simulink model "rfsocChannelizer"  (R2024a)
settings: Solver=FixedStepDiscrete  StartTime=0.0  StopTime=inf  RelTol=1e-3
InitFcn:
  | %% Polyphase Setup
  | fftsize = 512;
  | ntaps = 12;
  | vsize = 16;
  | pfb = dsp.Channelizer('NumFrequencyBands',fftsize,'NumTapsPerBand',ntaps);
  | 
  | coe = pfb.coeffs;
  | coe = coe.Numerator;
  | 
  | 
  | 
  | %% NCO Setup
  | rfsocChannelizerInit();
values from neighbouring files (symbols this model uses):
  Fo = 200.7e6    (= 200700000)    [rfsocChannelizerInit.m]
  Fs = 1/Ts    (= 5000000000)    [rfsocChannelizerInit.m]
  incrScale = (2^N)/Fs    (= 3.2768e-06)    [rfsocChannelizerInit.m]
  N = 14    [rfsocChannelizerInit.m]
libraries: dsphdlsigops2 x12, hdlsllib x9, simulink x8, simulink_need_slupdate x2, dspmathops x1, dsphdlfiltering2 x1, dspsrcs4 x1
Description:
  | libiioSDRPSP_filter_example
  | 
  | A simple example model to demonstrate the use of MATLAB I/O alongside
  | hardware/software co-design.
  | 
  | Implements AXI programmable gain and bypassable filters on the Tx and Rx
  | paths of the HDL DUT.
settings Model: DataTypeOverride=Off  ExtModeTrigDuration=100  Creator=mfornero  LastModifiedBy=versal
settings SolverCC: AlgebraicLoopSolver=TrustRegion  PositivePriorityOrder=on  MaxZcPerStep=1
settings DataIOCC: SaveOutput=off  ReturnWorkspaceOutputs=off  StateSaveName=tmp_raccel_xout  SignalLoggingName=tmp_raccel_logsout
settings OptimizationCC: BlockReduction=off  ConditionallyExecuteInputs=off  DefaultParameterBehavior=Inlined  EnhancedBackFolding=on  PassReuseOutputArgsAs=Individual arguments  ZeroExternalMemoryAtStartup=off  ZeroInternalMemoryAtStartup=off  EfficientMapNaN2IntZero=off  MaxStackSize=64  OptimizeBlockOrder=speed  DifferentSizesBufferReuse=on  OptimizationCustomize=off  EfficientTunableParamExpr=on
settings DebuggingCC: AlgebraicLoopMsg=error  SingleTaskRateTransMsg=error  ParameterTunabilityLossMsg=error  UnconnectedInputMsg=warning  UnconnectedOutputMsg=warning  UnconnectedLineMsg=warning  PregeneratedLibrarySubsystemCodeDiagnostic=none  StrictBusMsg=ErrorOnBusTreatedAsVector  SFUnexpectedBacktrackingDiag=warning  SFNoUnconditionalDefaultTransitionDiag=warning  SFExecutionAtInitializationDiag=none  ArithmeticOperatorsInVariantConditions=warning
settings HardwareCC: ProdBitPerPointer=32  ProdBitPerSizeT=32  ProdBitPerPtrDiffT=32  ProdLargestAtomicFloat=None  ProdIntDivRoundTo=Undefined  ProdEndianess=Unspecified  ProdWordSize=32  ProdHWDeviceType=ASIC/FPGA->ASIC/FPGA  TargetBitPerLong=64  TargetBitPerPointer=64  TargetBitPerSizeT=64  TargetBitPerPtrDiffT=64  TargetLongLongMode=on  TargetIntDivRoundTo=Zero  TargetEndianess=LittleEndian  TargetWordSize=64  TargetHWDeviceType=Custom Processor->MATLAB Host Computer  ProdEqTarget=off  HardwareBoardFeatureSet=SoCBlockset
settings ModelReferenceCC: EnableRefExpFcnMdlSchedulingChecks=on  ModelReferenceNumInstancesAllowed=Single
settings SFSimCC: SimUseLocalCustomCode=off  CustomCodeUndefinedFunction=UseInterfaceOnly
settings RTWCC: Description=Embedded Coder  SystemTargetFile=ert.tlc  HardwareBoard=Xilinx Zynq UltraScale+ RFSoC ZCU208 Evaluation Kit  TLCOptions="-aInlineSetEventsForThisBaseRateFcn=TLC_FALSE -aSuppressMultiTaskScheduler=TLC_FALSE  -aRateBasedStepFcn=0"  TemplateMakefile=ert_default_tmf  RTWVerbose=off  RTWUseLocalCustomCode=off  RTWUseSimCustomCode=on  Toolchain=Linaro AArch64 Linux v6.3.1  GPUComputeCapability=3.5  DLArmComputeVersion=19.05
settings CodeAppCC: ForceParamTrailComments=on  IgnoreCustomStorageClasses=off  MaxIdLength=128  OperatorAnnotations=on  SimulinkDataObjDesc=on  SFDataObjDesc=on  MangleLength=10  InsertBlockDesc=on
settings ERTTargetCC: InlinedParameterPlacement=NonHierarchical
settings ConfigComp: CovMetricSettings=dw  CovSaveCumulativeToWorkspaceVar=on  CovSaveSingleToWorkspaceVar=on  CovExternalEMLEnable=off

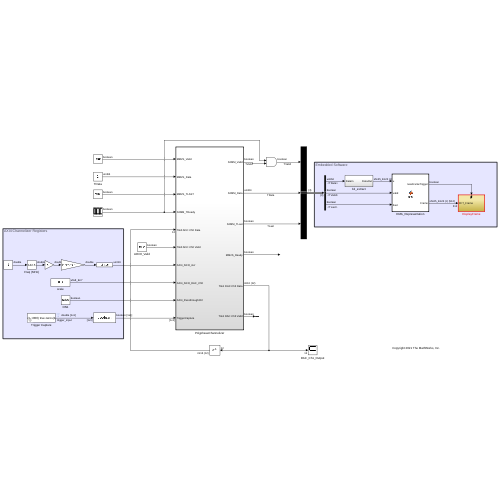
[thumbnail: Simulink's stored preview of the top-level diagram]
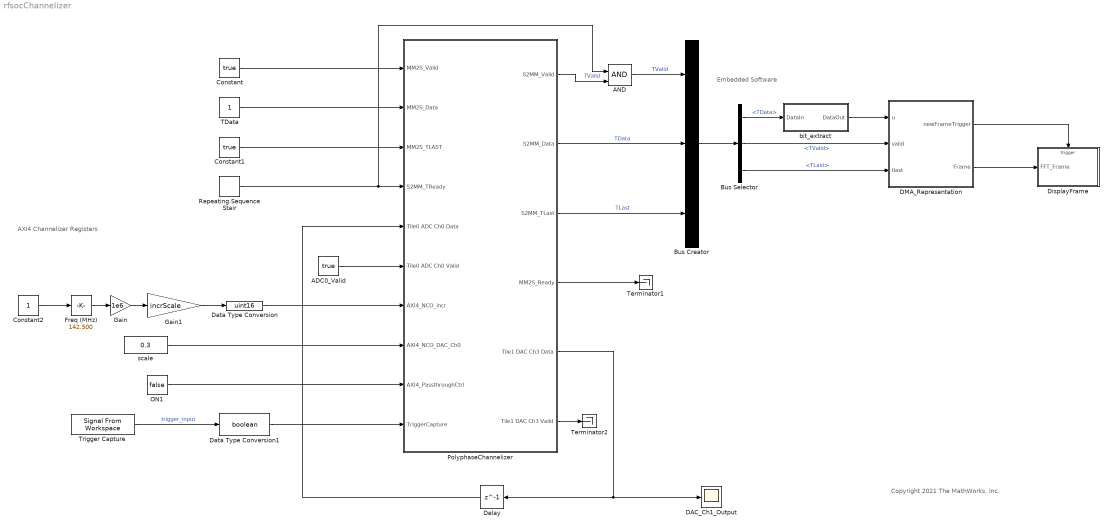
== system rfsocChannelizer ==
  note: AXI4 Channelizer Registers
  note: Embedded Software
  note: Copyright 2021 The MathWorks, Inc.
  ADC0_Valid : Constant  Value=true  SampleTime=-1
  AND : Logic  IconShape=distinctive  AllPortsSameDT=off  OutDataTypeStr=boolean
  Bus Creator : BusCreator  Inputs=3
  Bus Selector : BusSelector  OutputSignals=TData,TValid,TLast
  Constant : Constant  Value=true  SampleTime=1
  Constant1 : Constant  Value=true  SampleTime=-1
  Constant2 : Constant  SampleTime=1
  DAC_Ch1_Output : Scope
  DMA_Representation : MATLAB Function  TreatAsAtomicUnit=on
  Data Type Conversion : DataTypeConversion  OutDataTypeStr=uint16  SaturateOnIntegerOverflow=off  RndMeth=Floor
  Data Type Conversion1 : DataTypeConversion  OutDataTypeStr=boolean  SaturateOnIntegerOverflow=off  RndMeth=Floor
  Delay : Delay  DelayLength=1
  DisplayFrame : Subsystem
  Freq (MHz) : simulink/Math Operations/Slider Gain  gain=142.500  low=0  high=250
  Gain : Gain  Gain=1e6
  Gain1 : Gain  Gain=incrScale
  ON1 : Constant  Value=false  OutDataTypeStr=boolean  SampleTime=-1
  PolyphaseChannelizer : Subsystem  TreatAsAtomicUnit=on
  Repeating Sequence Stair : simulink/Sources/Repeating Sequence Stair  OutValues=[1 1 0 1 1 1 0 1 1]  tsamp=-1  OutMin=[]  OutMax=[]  OutDataTypeStr=fixdt('boolean')  OutputDataTypeScalingMode=Specify via dialog  OutDataType=fixdt('boolean')  ConRadixGroup=Best Precision: Vector-wise  OutScaling=[]
  TData : Constant  OutDataTypeStr=fixdt(0,64,0)  SampleTime=-1
  Terminator1 : Terminator
  Terminator2 : Terminator
  Trigger Capture : dspsrcs4/Signal From Workspace  X=[zeros(1,1000) true zeros(1,500)]  Ts=1  nsamps=1  OutputAfterFinalValue=Cyclic repetition  ignoreOrWarnInputAndFrameLengths=off  OutputFrames=off
  bit_extract : Subsystem
  scale : Constant  Value=0.3  OutDataTypeStr=fixdt(0,8,7)  SampleTime=-1
  wires:
  Constant/1 -> PolyphaseChannelizer/1(MM2S_Valid)
  TData/1 -> PolyphaseChannelizer/2(MM2S_Data)
  Gain/1 -> Gain1/1
  Freq (MHz)/1 -> Gain/1
  Constant2/1 -> Freq (MHz)/1
  Gain1/1 -> Data Type Conversion/1
  DMA_Representation/1(newFrameTrigger) -> DisplayFrame/Trigger
  DMA_Representation/2(Frame) -> DisplayFrame/1(FFT_Frame)
  bit_extract/1(DataOut) -> DMA_Representation/1(u)
  Constant1/1 -> PolyphaseChannelizer/3(MM2S_TLAST)
  PolyphaseChannelizer/4(MM2S_Ready) -> Terminator1/1
  Data Type Conversion/1 -> PolyphaseChannelizer/7(AXI4_NCO_incr)
  scale/1 -> PolyphaseChannelizer/8(AXI4_NCO_DAC_Ch0)
  ON1/1 -> PolyphaseChannelizer/9(AXI4_PassthroughCtrl)
  PolyphaseChannelizer/2(S2MM_Data) -> Bus Creator/2  "TData"
  PolyphaseChannelizer/3(S2MM_TLast) -> Bus Creator/3  "TLast"
  Bus Creator/1 -> Bus Selector/1
  Bus Selector/1 -> bit_extract/1(DataIn)  "<TData>"
  Bus Selector/2 -> DMA_Representation/2(valid)  "<TValid>"
  Bus Selector/3 -> DMA_Representation/3(tlast)  "<TLast>"
  ADC0_Valid/1 -> PolyphaseChannelizer/6(Tile0 ADC Ch0 Valid)
  PolyphaseChannelizer/6(Tile1 DAC Ch3 Valid) -> Terminator2/1
  PolyphaseChannelizer/5(Tile1 DAC Ch3 Data) -> Delay/1, DAC_Ch1_Output/1
  Trigger Capture/1 -> Data Type Conversion1/1  "trigger_input"
  Delay/1 -> PolyphaseChannelizer/5(Tile0 ADC Ch0 Data)
  Data Type Conversion1/1 -> PolyphaseChannelizer/10(TriggerCapture)
  PolyphaseChannelizer/1(S2MM_Valid) -> AND/2  "TValid"
  AND/1 -> Bus Creator/1  "TValid"
  Repeating Sequence Stair/1 -> AND/1, PolyphaseChannelizer/4(S2MM_TReady)

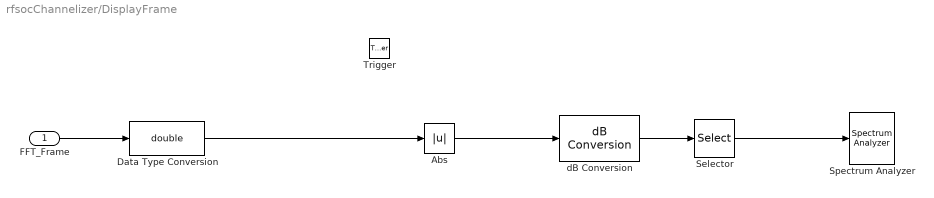
== system rfsocChannelizer/DisplayFrame ==
  FFT_Frame : Inport
  Trigger : TriggerPort  VariantControl=Variant
  Abs : Abs  SaturateOnIntegerOverflow=off
  Data Type Conversion : DataTypeConversion  OutDataTypeStr=double  SaturateOnIntegerOverflow=off  RndMeth=Floor
  Selector : Selector  InputPortWidth=512  IndexOptions=Index vector (dialog)  Indices=1:256  OutputSizes=1
  Spectrum Analyzer : SpectrumAnalyzer  WindowPosition=[613.000000,47.000000,1109.000000,792.000000,]  ScopeFrameLocation=window  InputDomain=Frequency  ViewType=Spectrum and spectrogram  SampleRateSource=Property  SampleRate=Fs  PlotAsTwoSidedSpectrum=off  AxesScaling=Manual  AveragingMethod=Exponential  SpectrumUnits=Auto  YLimits=[-140.0,0.1]  AllowFFTLengthLessThanSamplesPerUpdate=on  IsFrequencyInputMode=1
  dB Conversion : dspmathops/dB Conversion  dBtype=dB  intype=Amplitude  R=1  fuzz=on
  wires:
  FFT_Frame/1 -> Data Type Conversion/1
  dB Conversion/1 -> Selector/1
  Abs/1 -> dB Conversion/1
  Data Type Conversion/1 -> Abs/1
  Selector/1 -> Spectrum Analyzer/1

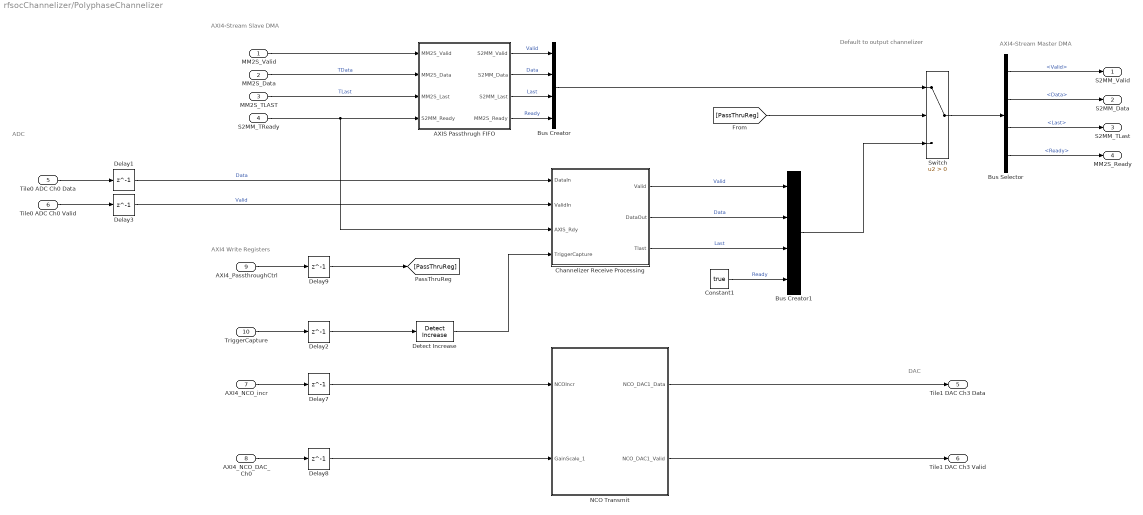
== system rfsocChannelizer/PolyphaseChannelizer ==
  note: Default to output channelizer
  note: DAC
  note: AXI4-Stream Slave DMA
  note: AXI4-Stream Master DMA
  note: AXI4 Write Registers
  note: ADC
  MM2S_Valid : Inport
  MM2S_Data : Inport  Port=2
  MM2S_TLAST : Inport  Port=3
  S2MM_TReady : Inport  Port=4
  Tile0 ADC Ch0 Data : Inport  Port=5
  Tile0 ADC Ch0 Valid : Inport  Port=6
  AXI4_NCO_incr : Inport  Port=7
  AXI4_NCO_DAC_Ch0 : Inport  Port=8
  AXI4_PassthroughCtrl : Inport  Port=9
  TriggerCapture : Inport  Port=10
  AXIS Passthrugh FIFO : Subsystem
  Bus Creator : BusCreator  Inputs=4
  Bus Creator1 : BusCreator  Inputs=4
  Bus Selector : BusSelector  OutputSignals=Valid,Data,Last,Ready
  "Channelizer Receive Processing " : Subsystem
  Constant1 : Constant  Value=true  OutDataTypeStr=boolean  SampleTime=-1
  Delay{1..3,7..9} (6 alike) : Delay  DelayLength=1
  Detect Increase : simulink/Logic and Bit Operations/Detect Increase  vinit=0.0  OutDataTypeStr=boolean
  NCO Transmit : Subsystem
  Switch : Switch  Criteria=u2 > Threshold  SaturateOnIntegerOverflow=off  InputSameDT=off
  S2MM_Valid : Outport  VectorParamsAs1DForOutWhenUnconnected=off
  S2MM_Data : Outport  Port=2  VectorParamsAs1DForOutWhenUnconnected=off
  S2MM_TLast : Outport  Port=3  VectorParamsAs1DForOutWhenUnconnected=off
  MM2S_Ready : Outport  Port=4  VectorParamsAs1DForOutWhenUnconnected=off
  Tile1 DAC Ch3 Data : Outport  Port=5
  Tile1 DAC Ch3 Valid : Outport  Port=6
  wires:
  Tile0 ADC Ch0 Data/1 -> Delay1/1
  Tile0 ADC Ch0 Valid/1 -> Delay3/1
  MM2S_Data/1 -> AXIS Passthrugh FIFO/2(MM2S_Data)  "TData"
  S2MM_TReady/1 -> AXIS Passthrugh FIFO/4(S2MM_Ready), "Channelizer Receive Processing "/3(AXIS_Rdy)
  "Channelizer Receive Processing "/3(Tlast) -> Bus Creator1/3  "Last"
  Bus Selector/4 -> MM2S_Ready/1  "<Ready>"
  AXI4_NCO_incr/1 -> Delay7/1
  AXI4_NCO_DAC_Ch0/1 -> Delay8/1
  NCO Transmit/1(NCO_DAC1_Data) -> Tile1 DAC Ch3 Data/1
  NCO Transmit/2(NCO_DAC1_Valid) -> Tile1 DAC Ch3 Valid/1
  MM2S_TLAST/1 -> AXIS Passthrugh FIFO/3(MM2S_Last)  "TLast"
  AXI4_PassthroughCtrl/1 -> Delay9/1
  Delay9/1 -> [PassThruReg]
  [PassThruReg] -> Switch/2
  "Channelizer Receive Processing "/2(DataOut) -> Bus Creator1/2  "Data"
  "Channelizer Receive Processing "/1(Valid) -> Bus Creator1/1  "Valid"
  Bus Creator1/1 -> Switch/3
  Bus Selector/1 -> S2MM_Valid/1  "<Valid>"
  Bus Selector/2 -> S2MM_Data/1  "<Data>"
  Bus Selector/3 -> S2MM_TLast/1  "<Last>"
  MM2S_Valid/1 -> AXIS Passthrugh FIFO/1(MM2S_Valid)
  AXIS Passthrugh FIFO/4(MM2S_Ready) -> Bus Creator/4  "Ready"
  AXIS Passthrugh FIFO/3(S2MM_Last) -> Bus Creator/3  "Last"
  AXIS Passthrugh FIFO/2(S2MM_Data) -> Bus Creator/2  "Data"
  AXIS Passthrugh FIFO/1(S2MM_Valid) -> Bus Creator/1  "Valid"
  Bus Creator/1 -> Switch/1
  Constant1/1 -> Bus Creator1/4  "Ready"
  Switch/1 -> Bus Selector/1
  Delay3/1 -> "Channelizer Receive Processing "/2(ValidIn)  "Valid"
  Delay1/1 -> "Channelizer Receive Processing "/1(DataIn)  "Data"
  Delay7/1 -> NCO Transmit/1(NCOIncr)
  Delay8/1 -> NCO Transmit/2(GainScale_1)
  TriggerCapture/1 -> Delay2/1
  Delay2/1 -> Detect Increase/1
  Detect Increase/1 -> "Channelizer Receive Processing "/4(TriggerCapture)

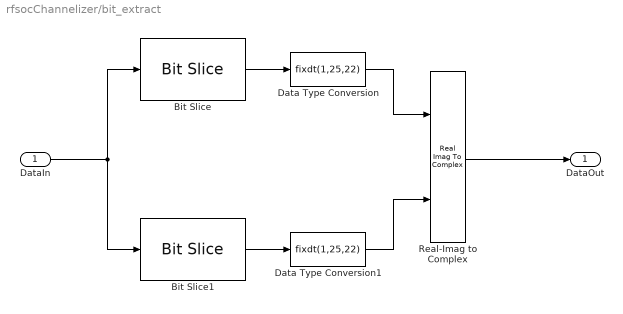
== system rfsocChannelizer/bit_extract ==
  DataIn : Inport
  Bit Slice : hdlsllib/Logic and Bit Operations/Bit Slice  lidx=49  ridx=25
  Bit Slice1 : hdlsllib/Logic and Bit Operations/Bit Slice  lidx=24  ridx=0
  Data Type Conversion : DataTypeConversion  OutDataTypeStr=fixdt(1,25,22)  ConvertRealWorld=Stored Integer (SI)  SaturateOnIntegerOverflow=off  RndMeth=Floor
  Data Type Conversion1 : DataTypeConversion  OutDataTypeStr=fixdt(1,25,22)  ConvertRealWorld=Stored Integer (SI)  SaturateOnIntegerOverflow=off  RndMeth=Floor
  Real-Imag to Complex : RealImagToComplex
  DataOut : Outport  VectorParamsAs1DForOutWhenUnconnected=off
  wires:
  DataIn/1 -> Bit Slice1/1, Bit Slice/1
  Bit Slice/1 -> Data Type Conversion/1
  Bit Slice1/1 -> Data Type Conversion1/1
  Data Type Conversion/1 -> Real-Imag to Complex/1
  Data Type Conversion1/1 -> Real-Imag to Complex/2
  Real-Imag to Complex/1 -> DataOut/1

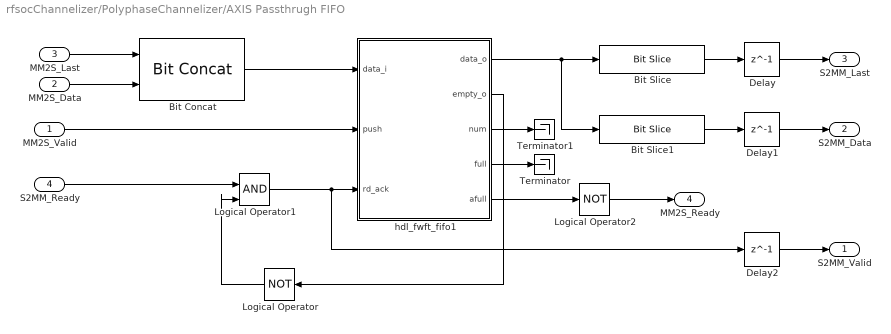
== system rfsocChannelizer/PolyphaseChannelizer/AXIS Passthrugh FIFO ==
  MM2S_Valid : Inport
  MM2S_Data : Inport  Port=2
  MM2S_Last : Inport  Port=3
  S2MM_Ready : Inport  Port=4
  Bit Concat : hdlsllib/Logic and Bit Operations/Bit Concat  numInputs=2
  Bit Slice : hdlsllib/Logic and Bit Operations/Bit Slice  lidx=64  ridx=64
  Bit Slice1 : hdlsllib/Logic and Bit Operations/Bit Slice  lidx=63  ridx=0
  Delay : Delay  DelayLength=1
  Delay1 : Delay  DelayLength=1
  Delay2 : Delay  DelayLength=1
  Logical Operator : Logic  Operator=NOT  IconShape=distinctive  AllPortsSameDT=off  OutDataTypeStr=boolean
  Logical Operator1 : Logic  IconShape=distinctive  AllPortsSameDT=off  OutDataTypeStr=boolean
  Logical Operator2 : Logic  Operator=NOT  IconShape=distinctive  AllPortsSameDT=off  OutDataTypeStr=boolean
  Terminator : Terminator
  Terminator1 : Terminator
  hdl_fwft_fifo1 : Subsystem  mask{FIFO_DEPTH=100, AFULL_THRESH=80}
      mask prompts: FIFO_DEPTH "FIFO Depth"; AFULL_THRESH "Almost Full Threshold"
      mask init:
      | FIFO_CNT_BITS=ceil(log2(FIFO_DEPTH+1+3));
  S2MM_Valid : Outport  VectorParamsAs1DForOutWhenUnconnected=off
  S2MM_Data : Outport  Port=2  VectorParamsAs1DForOutWhenUnconnected=off
  S2MM_Last : Outport  Port=3  VectorParamsAs1DForOutWhenUnconnected=off
  MM2S_Ready : Outport  Port=4  VectorParamsAs1DForOutWhenUnconnected=off
  wires:
  MM2S_Data/1 -> Bit Concat/2
  Bit Concat/1 -> hdl_fwft_fifo1/1(data_i)
  MM2S_Last/1 -> Bit Concat/1
  Logical Operator1/1 -> Delay2/1, hdl_fwft_fifo1/3(rd_ack)
  hdl_fwft_fifo1/2(empty_o) -> Logical Operator/1
  S2MM_Ready/1 -> Logical Operator1/1
  Bit Slice/1 -> Delay/1
  hdl_fwft_fifo1/1(data_o) -> Bit Slice1/1, Bit Slice/1
  Logical Operator/1 -> Logical Operator1/2
  hdl_fwft_fifo1/4(full) -> Terminator/1
  Delay2/1 -> S2MM_Valid/1
  Delay/1 -> S2MM_Last/1
  hdl_fwft_fifo1/3(num) -> Terminator1/1
  Delay1/1 -> S2MM_Data/1
  hdl_fwft_fifo1/5(afull) -> Logical Operator2/1
  Logical Operator2/1 -> MM2S_Ready/1
  Bit Slice1/1 -> Delay1/1
  MM2S_Valid/1 -> hdl_fwft_fifo1/2(push)

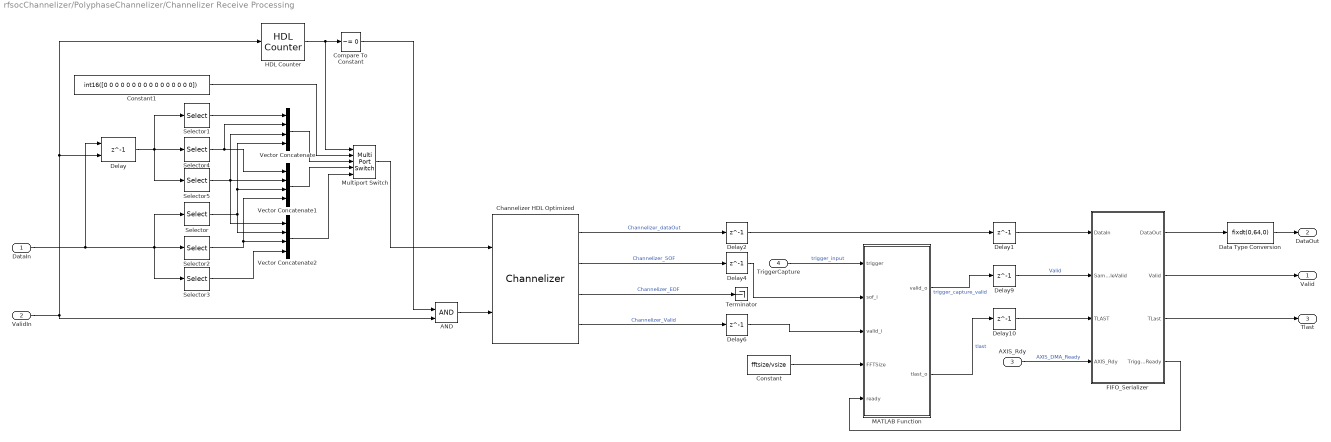
== system rfsocChannelizer/PolyphaseChannelizer/Channelizer Receive Processing  ==
  DataIn : Inport
  ValidIn : Inport  Port=2
  AXIS_Rdy : Inport  Port=3
  TriggerCapture : Inport  Port=4
  AND : Logic  IconShape=distinctive  AllPortsSameDT=off  OutDataTypeStr=boolean
  Channelizer HDL Optimized : dsphdlfiltering2/Channelizer  FilterCoefficients=pfb.coeffs.Numerator  FilterStructure=Direct form transposed  NumFrequencyBands=fftsize  ComplexMultiplication=Use 3 multipliers and 5 adders  Normalize=off  OutputSize=Same as input size  SimulateUsing=Code generation  roundingMode=Floor  overflowMode=off  CoefficientsDataTypeStr=Inherit: Same word length as input  FilterOutputDataTypeStr=Inherit: Same word length as input  ResetInputPort=off  StartOutputPort=on  EndOutputPort=on
  Compare To Constant : simulink/Logic and Bit Operations/Compare To Constant  relop=~=  const=0  OutDataTypeStr=boolean
  Constant : Constant  Value=fftsize/vsize  OutDataTypeStr=uint16  SampleTime=-1
  Constant1 : Constant  Value=int16([0 0 0 0 0 0 0 0 0 0 0 0 0 0 0 0])
  Data Type Conversion : DataTypeConversion  OutDataTypeStr=fixdt(0,64,0)  ConvertRealWorld=Stored Integer (SI)  SaturateOnIntegerOverflow=off  RndMeth=Floor
  Delay : Delay  DelayLength=1  InitialCondition=0  ShowEnablePort=on  UseCircularBuffer=on
      settings: InputPortMap=u0,e6
  Delay{1..2,4,6,9..10} (6 alike) : Delay  DelayLength=1
  FIFO_Serializer : Subsystem
  HDL Counter : hdlsllib/Sources/HDL Counter  CountType=Count limited  CountInit=0  CountStep=1  CountMax=3  CountFromType=Initial value  CountFrom=0  CountResetPort=off  CountLoadPort=off  CountEnbPort=on  CountDirPort=off  CountHitOutputPort=off  CountDataType=Unsigned  CountWordLen=2  CountFracLen=0  CountSampTime=1
  MATLAB Function : MATLAB Function  TreatAsAtomicUnit=on
  Multiport Switch : MultiPortSwitch  DataPortOrder=Zero-based contiguous  Inputs=4  zeroidx=on  SaturateOnIntegerOverflow=off  InputSameDT=off
  Selector : Selector  InputPortWidth=12  IndexOptions=Index vector (dialog)  Indices=[1 2 3 4]  OutputSizes=1
  Selector1 : Selector  InputPortWidth=12  IndexOptions=Index vector (dialog)  Indices=[1 2 3 4]  OutputSizes=1
  Selector2 : Selector  InputPortWidth=12  IndexOptions=Index vector (dialog)  Indices=[5 6 7 8]  OutputSizes=1
  Selector3 : Selector  InputPortWidth=12  IndexOptions=Index vector (dialog)  Indices=[9 10 11 12]  OutputSizes=1
  Selector4 : Selector  InputPortWidth=12  IndexOptions=Index vector (dialog)  Indices=[5 6 7 8]  OutputSizes=1
  Selector5 : Selector  InputPortWidth=12  IndexOptions=Index vector (dialog)  Indices=[9 10 11 12]  OutputSizes=1
  Terminator : Terminator
  Vector Concatenate : Concatenate  NumInputs=4
  Vector Concatenate1 : Concatenate  NumInputs=4
  Vector Concatenate2 : Concatenate  NumInputs=4
  Valid : Outport  VectorParamsAs1DForOutWhenUnconnected=off
  DataOut : Outport  Port=2  VectorParamsAs1DForOutWhenUnconnected=off
  Tlast : Outport  Port=3  VectorParamsAs1DForOutWhenUnconnected=off
  wires:
  Delay9/1 -> FIFO_Serializer/2(SampleValid)  "Valid"
  Delay10/1 -> FIFO_Serializer/3(TLAST)
  Delay1/1 -> FIFO_Serializer/1(DataIn)
  AXIS_Rdy/1 -> FIFO_Serializer/4(AXIS_Rdy)  "AXIS_DMA_Ready"
  FIFO_Serializer/1(DataOut) -> Data Type Conversion/1
  Data Type Conversion/1 -> DataOut/1
  FIFO_Serializer/2(Valid) -> Valid/1
  ValidIn/1 -> Delay/2, HDL Counter/1, AND/2
  Channelizer HDL Optimized/1 -> Delay2/1  "Channelizer_dataOut"
  Channelizer HDL Optimized/2 -> Delay4/1  "Channelizer_SOF"
  Channelizer HDL Optimized/3 -> Terminator/1  "Channelizer_EOF"
  Channelizer HDL Optimized/4 -> Delay6/1  "Channelizer_Valid"
  FIFO_Serializer/3(TLast) -> Tlast/1
  Constant/1 -> MATLAB Function/4(FFTSize)
  FIFO_Serializer/4(TriggerReady) -> MATLAB Function/5(ready)
  TriggerCapture/1 -> MATLAB Function/1(trigger)  "trigger_input"
  MATLAB Function/1(valid_o) -> Delay9/1  "trigger_capture_valid"
  Delay4/1 -> MATLAB Function/2(sof_i)
  Delay6/1 -> MATLAB Function/3(valid_i)
  MATLAB Function/2(tlast_o) -> Delay10/1  "tlast"
  Delay2/1 -> Delay1/1
  DataIn/1 -> Selector3/1, Selector2/1, Selector/1, Delay/1
  Delay/1 -> Selector4/1, Selector5/1, Selector1/1
  Selector1/1 -> Vector Concatenate/1
  Selector4/1 -> Vector Concatenate1/1, Vector Concatenate/2
  Selector5/1 -> Vector Concatenate2/1, Vector Concatenate1/2, Vector Concatenate/3
  Selector/1 -> Vector Concatenate1/3, Vector Concatenate/4, Vector Concatenate2/2
  Selector2/1 -> Vector Concatenate2/3, Vector Concatenate1/4
  Selector3/1 -> Vector Concatenate2/4
  Vector Concatenate/1 -> Multiport Switch/3
  Vector Concatenate1/1 -> Multiport Switch/4
  Vector Concatenate2/1 -> Multiport Switch/5
  Multiport Switch/1 -> Channelizer HDL Optimized/1
  HDL Counter/1 -> Compare To Constant/1, Multiport Switch/1
  Constant1/1 -> Multiport Switch/2
  AND/1 -> Channelizer HDL Optimized/2
  Compare To Constant/1 -> AND/1

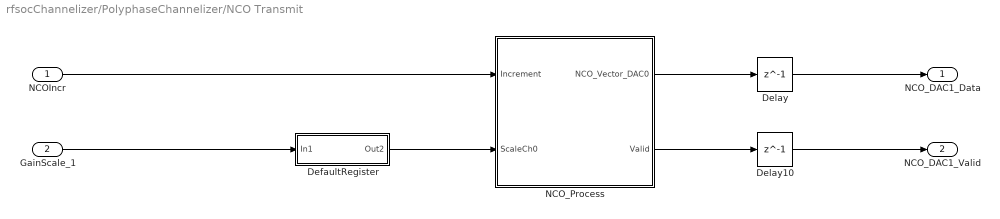
== system rfsocChannelizer/PolyphaseChannelizer/NCO Transmit ==
  NCOIncr : Inport
  GainScale_1 : Inport  Port=2
  DefaultRegister : Subsystem
  Delay : Delay  DelayLength=1
  Delay10 : Delay  DelayLength=1
  NCO_Process : Subsystem
  NCO_DAC1_Data : Outport  VectorParamsAs1DForOutWhenUnconnected=off
  NCO_DAC1_Valid : Outport  Port=2  VectorParamsAs1DForOutWhenUnconnected=off
  wires:
  Delay/1 -> NCO_DAC1_Data/1
  DefaultRegister/1(Out2) -> NCO_Process/2(ScaleCh0)
  NCO_Process/1(NCO_Vector_DAC0) -> Delay/1
  NCO_Process/2(Valid) -> Delay10/1
  NCOIncr/1 -> NCO_Process/1(Increment)
  GainScale_1/1 -> DefaultRegister/1(In1)
  Delay10/1 -> NCO_DAC1_Valid/1

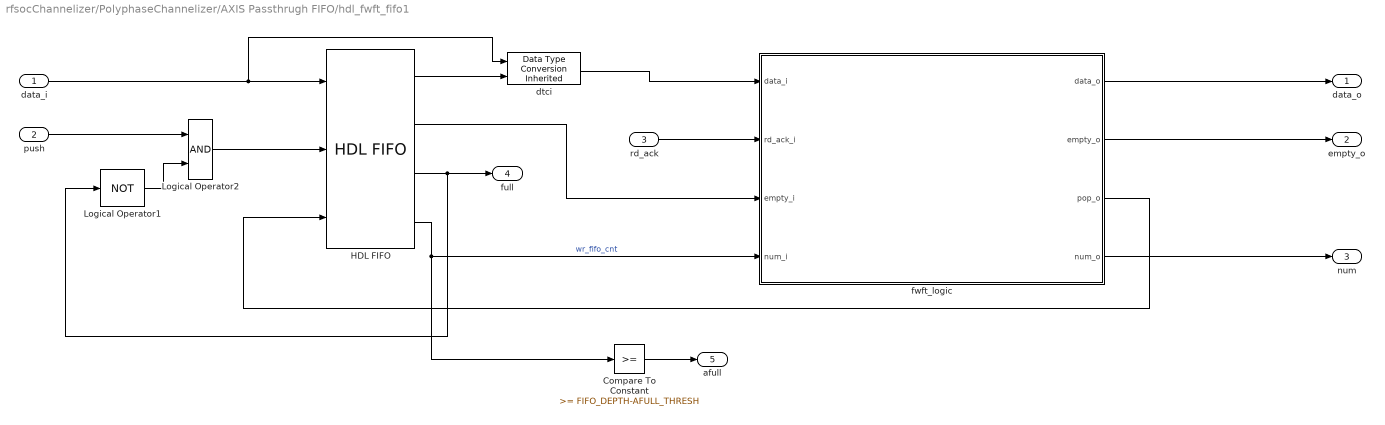
== system rfsocChannelizer/PolyphaseChannelizer/AXIS Passthrugh FIFO/hdl_fwft_fifo1 ==
  data_i : Inport
  push : Inport  Port=2
  rd_ack : Inport  Port=3
  Compare To Constant : simulink/Logic and Bit Operations/Compare To Constant  relop=>=  const=FIFO_DEPTH-AFULL_THRESH  OutDataTypeStr=boolean
  HDL FIFO : hdlsllib/HDL RAMs/HDL FIFO  fifo_size=FIFO_DEPTH  mode=Classic  ratio=1  push_msg=Error  pop_msg=Ignore  show_empty=on  show_full=on  show_num=on  LabelModeActiveChoice_Mode=Classic  rst_port=off
  Logical Operator1 : Logic  Operator=NOT  IconShape=distinctive  AllPortsSameDT=off  OutDataTypeStr=boolean
  Logical Operator2 : Logic  IconShape=distinctive  AllPortsSameDT=off  OutDataTypeStr=boolean
  dtci : simulink/Signal Attributes/Data Type Conversion Inherited  ConvertRealWorld=Real World Value  DoSatur=off
  fwft_logic : Subsystem
  data_o : Outport  VectorParamsAs1DForOutWhenUnconnected=off
  empty_o : Outport  Port=2  VectorParamsAs1DForOutWhenUnconnected=off
  num : Outport  Port=3  VectorParamsAs1DForOutWhenUnconnected=off
  full : Outport  Port=4  VectorParamsAs1DForOutWhenUnconnected=off
  afull : Outport  Port=5  VectorParamsAs1DForOutWhenUnconnected=off
  wires:
  Compare To Constant/1 -> afull/1
  fwft_logic/1(data_o) -> data_o/1
  HDL FIFO/2 -> fwft_logic/3(empty_i)
  rd_ack/1 -> fwft_logic/2(rd_ack_i)
  fwft_logic/2(empty_o) -> empty_o/1
  data_i/1 -> dtci/1, HDL FIFO/1
  fwft_logic/3(pop_o) -> HDL FIFO/3
  push/1 -> Logical Operator2/1
  Logical Operator2/1 -> HDL FIFO/2
  Logical Operator1/1 -> Logical Operator2/2
  HDL FIFO/1 -> dtci/2
  dtci/1 -> fwft_logic/1(data_i)
  HDL FIFO/3 -> Logical Operator1/1, full/1
  HDL FIFO/4 -> Compare To Constant/1, fwft_logic/4(num_i)  "wr_fifo_cnt"
  fwft_logic/4(num_o) -> num/1

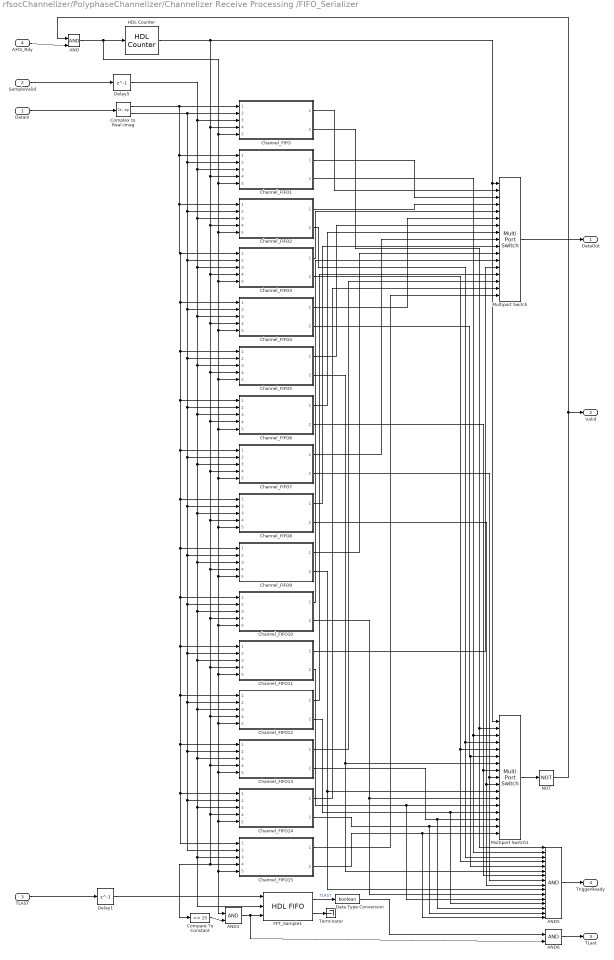
== system rfsocChannelizer/PolyphaseChannelizer/Channelizer Receive Processing /FIFO_Serializer ==
  DataIn : Inport
  SampleValid : Inport  Port=2
  TLAST : Inport  Port=3
  AXIS_Rdy : Inport  Port=4
  AND : Logic  IconShape=distinctive  AllPortsSameDT=off  OutDataTypeStr=boolean
  AND1 : Logic  IconShape=distinctive  AllPortsSameDT=off  OutDataTypeStr=boolean
  AND5 : Logic  Inputs=16  IconShape=distinctive  AllPortsSameDT=off  OutDataTypeStr=boolean
  AND6 : Logic  IconShape=distinctive  AllPortsSameDT=off  OutDataTypeStr=boolean
  Channel_FIFO : Subsystem  ReferencedSubsystem=Channel_FIFO  Index=0
  Channel_FIFO1 : Subsystem  ReferencedSubsystem=Channel_FIFO  Index=1
  Channel_FIFO10 : Subsystem  ReferencedSubsystem=Channel_FIFO  Index=10
  Channel_FIFO11 : Subsystem  ReferencedSubsystem=Channel_FIFO  Index=11
  Channel_FIFO12 : Subsystem  ReferencedSubsystem=Channel_FIFO  Index=12
  Channel_FIFO13 : Subsystem  ReferencedSubsystem=Channel_FIFO  Index=13
  Channel_FIFO14 : Subsystem  ReferencedSubsystem=Channel_FIFO  Index=14
  Channel_FIFO15 : Subsystem  ReferencedSubsystem=Channel_FIFO  Index=15
  Channel_FIFO2 : Subsystem  ReferencedSubsystem=Channel_FIFO  Index=2
  Channel_FIFO3 : Subsystem  ReferencedSubsystem=Channel_FIFO  Index=3
  Channel_FIFO4 : Subsystem  ReferencedSubsystem=Channel_FIFO  Index=4
  Channel_FIFO5 : Subsystem  ReferencedSubsystem=Channel_FIFO  Index=5
  Channel_FIFO6 : Subsystem  ReferencedSubsystem=Channel_FIFO  Index=6
  Channel_FIFO7 : Subsystem  ReferencedSubsystem=Channel_FIFO  Index=7
  Channel_FIFO8 : Subsystem  ReferencedSubsystem=Channel_FIFO  Index=8
  Channel_FIFO9 : Subsystem  ReferencedSubsystem=Channel_FIFO  Index=9
  Compare To Constant : simulink/Logic and Bit Operations/Compare To Constant  relop===  const=15  OutDataTypeStr=boolean
  Complex to Real-Imag : ComplexToRealImag
  Data Type Conversion : DataTypeConversion  OutDataTypeStr=boolean  SaturateOnIntegerOverflow=off  RndMeth=Floor
  Delay1 : Delay  DelayLength=1
  Delay5 : Delay  DelayLength=1
  FFT_Sample1 : hdlsllib/HDL RAMs/HDL FIFO  fifo_size=128  mode=FWFT  ratio=1  push_msg=Warning  pop_msg=Warning  show_empty=on  show_full=off  show_num=off  LabelModeActiveChoice_Mode=FWFT  rst_port=off
  HDL Counter : hdlsllib/Sources/HDL Counter  CountType=Count limited  CountInit=0  CountStep=1  CountMax=15  CountFromType=Initial value  CountFrom=0  CountResetPort=off  CountLoadPort=off  CountEnbPort=on  CountDirPort=off  CountHitOutputPort=off  CountDataType=Unsigned  CountWordLen=4  CountFracLen=0  CountSampTime=1
  Multiport Switch : MultiPortSwitch  DataPortOrder=Zero-based contiguous  Inputs=16  zeroidx=on  SaturateOnIntegerOverflow=off  InputSameDT=off
  Multiport Switch1 : MultiPortSwitch  DataPortOrder=Zero-based contiguous  Inputs=16  zeroidx=on  SaturateOnIntegerOverflow=off  InputSameDT=off
  NOT : Logic  Operator=NOT  IconShape=distinctive  AllPortsSameDT=off  OutDataTypeStr=boolean
  Terminator : Terminator
  DataOut : Outport  VectorParamsAs1DForOutWhenUnconnected=off
  Valid : Outport  Port=2  VectorParamsAs1DForOutWhenUnconnected=off
  TLast : Outport  Port=3  VectorParamsAs1DForOutWhenUnconnected=off
  TriggerReady : Outport  Port=4
  wires:
  AND1/1 -> AND6/2, FFT_Sample1/3
  Channel_FIFO2/1 -> Multiport Switch/4
  Compare To Constant/1 -> AND1/2
  DataIn/1 -> Complex to Real-Imag/1
  Data Type Conversion/1 -> AND6/1
  Channel_FIFO2/2 -> AND5/3, Multiport Switch1/4
  Channel_FIFO/1 -> Multiport Switch/2
  Multiport Switch/1 -> DataOut/1
  TLAST/1 -> Delay1/1
  Channel_FIFO1/1 -> Multiport Switch/3
  NOT/1 -> AND/1, Valid/1
  FFT_Sample1/1 -> Data Type Conversion/1  "TLAST"
  Channel_FIFO1/2 -> AND5/2, Multiport Switch1/3
  AXIS_Rdy/1 -> AND/2
  SampleValid/1 -> Delay5/1
  AND6/1 -> TLast/1
  Channel_FIFO/2 -> AND5/1, Multiport Switch1/2
  AND5/1 -> TriggerReady/1
  Channel_FIFO3/2 -> AND5/4, Multiport Switch1/5
  Multiport Switch1/1 -> NOT/1
  Channel_FIFO3/1 -> Multiport Switch/5
  Complex to Real-Imag/1 -> Channel_FIFO1/1, Channel_FIFO2/1, Channel_FIFO3/1, Channel_FIFO4/1, Channel_FIFO5/1, Channel_FIFO6/1, Channel_FIFO7/1, Channel_FIFO8/1, Channel_FIFO9/1, Channel_FIFO10/1, Channel_FIFO11/1, Channel_FIFO12/1, Channel_FIFO13/1, Channel_FIFO14/1, Channel_FIFO15/1, Channel_FIFO/1
  Complex to Real-Imag/2 -> Channel_FIFO1/2, Channel_FIFO2/2, Channel_FIFO3/2, Channel_FIFO4/2, Channel_FIFO5/2, Channel_FIFO6/2, Channel_FIFO7/2, Channel_FIFO8/2, Channel_FIFO9/2, Channel_FIFO10/2, Channel_FIFO11/2, Channel_FIFO12/2, Channel_FIFO13/2, Channel_FIFO14/2, Channel_FIFO15/2, Channel_FIFO/2
  AND/1 -> Channel_FIFO1/5, Channel_FIFO2/5, Channel_FIFO3/5, Channel_FIFO4/5, Channel_FIFO5/5, Channel_FIFO6/5, Channel_FIFO7/5, Channel_FIFO8/5, Channel_FIFO9/5, Channel_FIFO10/5, Channel_FIFO11/5, Channel_FIFO12/5, Channel_FIFO13/5, Channel_FIFO14/5, Channel_FIFO15/5, AND1/1, Channel_FIFO/5, HDL Counter/1
  Delay5/1 -> Channel_FIFO1/3, Channel_FIFO2/3, FFT_Sample1/2, Channel_FIFO15/3, Channel_FIFO14/3, Channel_FIFO13/3, Channel_FIFO12/3, Channel_FIFO11/3, Channel_FIFO10/3, Channel_FIFO9/3, Channel_FIFO8/3, Channel_FIFO7/3, Channel_FIFO6/3, Channel_FIFO5/3, Channel_FIFO4/3, Channel_FIFO3/3, Channel_FIFO/3
  Channel_FIFO4/1 -> Multiport Switch/6
  Channel_FIFO5/1 -> Multiport Switch/7
  Channel_FIFO6/1 -> Multiport Switch/8
  Channel_FIFO7/1 -> Multiport Switch/9
  Channel_FIFO8/1 -> Multiport Switch/10
  Channel_FIFO9/1 -> Multiport Switch/11
  Channel_FIFO10/1 -> Multiport Switch/12
  Channel_FIFO11/1 -> Multiport Switch/13
  Channel_FIFO12/1 -> Multiport Switch/14
  Channel_FIFO13/1 -> Multiport Switch/15
  Channel_FIFO14/1 -> Multiport Switch/16
  Channel_FIFO15/1 -> Multiport Switch/17
  Channel_FIFO4/2 -> AND5/5, Multiport Switch1/6
  Channel_FIFO5/2 -> AND5/6, Multiport Switch1/7
  Channel_FIFO7/2 -> AND5/8, Multiport Switch1/9
  Channel_FIFO8/2 -> AND5/9, Multiport Switch1/10
  Channel_FIFO9/2 -> AND5/10, Multiport Switch1/11
  Channel_FIFO10/2 -> AND5/11, Multiport Switch1/12
  Channel_FIFO11/2 -> AND5/12, Multiport Switch1/13
  Channel_FIFO12/2 -> AND5/13, Multiport Switch1/14
  Channel_FIFO13/2 -> AND5/14, Multiport Switch1/15
  Channel_FIFO14/2 -> AND5/15, Multiport Switch1/16
  Channel_FIFO15/2 -> AND5/16, Multiport Switch1/17
  Channel_FIFO6/2 -> AND5/7, Multiport Switch1/8
  FFT_Sample1/2 -> Terminator/1
  Delay1/1 -> FFT_Sample1/1
  HDL Counter/1 -> Multiport Switch/1, Multiport Switch1/1, Channel_FIFO1/4, Channel_FIFO2/4, Channel_FIFO3/4, Channel_FIFO4/4, Channel_FIFO5/4, Channel_FIFO6/4, Channel_FIFO7/4, Channel_FIFO8/4, Channel_FIFO9/4, Channel_FIFO10/4, Channel_FIFO11/4, Channel_FIFO12/4, Channel_FIFO13/4, Channel_FIFO14/4, Channel_FIFO15/4, Compare To Constant/1, Channel_FIFO/4

== system rfsocChannelizer/PolyphaseChannelizer/NCO Transmit/DefaultRegister ==
  note: Give it default non-zero value at start-up time
  In1 : Inport
  Compare To Zero : simulink/Logic and Bit Operations/Compare To Zero  relop===  OutDataTypeStr=boolean
  Constant5 : Constant  Value=0.3  OutDataTypeStr=fixdt(0,4,4)  SampleTime=-1
  Delay1 : Delay  DelayLength=1
  Switch2 : Switch  Criteria=u2 > Threshold  SaturateOnIntegerOverflow=off  InputSameDT=off
  Out2 : Outport  VectorParamsAs1DForOutWhenUnconnected=off
  wires:
  In1/1 -> Delay1/1
  Constant5/1 -> Switch2/1
  Delay1/1 -> Switch2/3, Compare To Zero/1
  Switch2/1 -> Out2/1
  Compare To Zero/1 -> Switch2/2

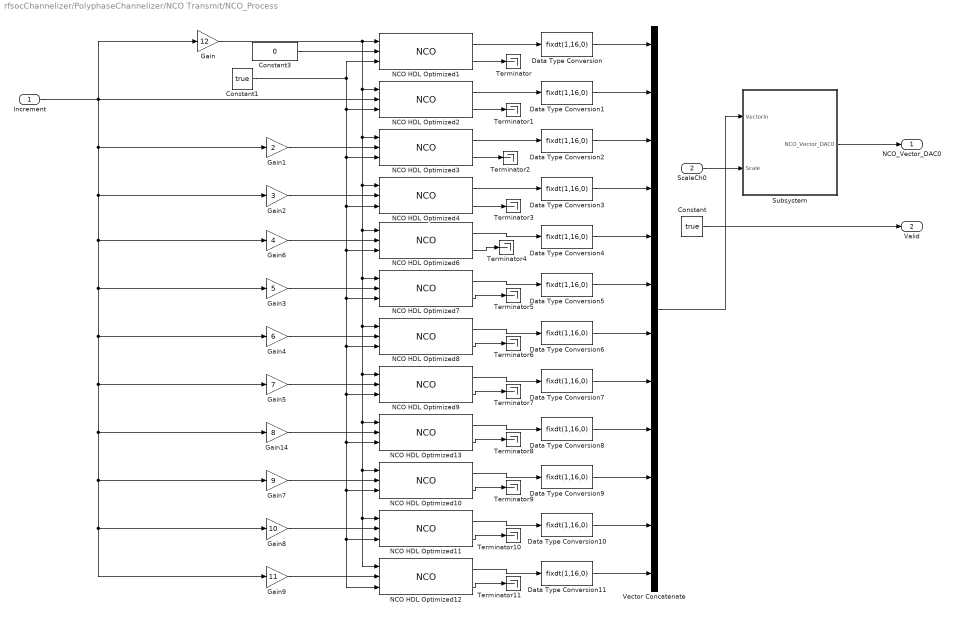
== system rfsocChannelizer/PolyphaseChannelizer/NCO Transmit/NCO_Process ==
  Increment : Inport
  ScaleCh0 : Inport  Port=2
  Constant : Constant  Value=true  SampleTime=-1
  Constant1 : Constant  Value=true  SampleTime=-1
  Constant3 : Constant  Value=0  OutDataTypeStr=uint16  SampleTime=-1
  Data Type Conversion{,1..11} (12 alike) : DataTypeConversion  OutDataTypeStr=fixdt(1,16,0)  ConvertRealWorld=Stored Integer (SI)  SaturateOnIntegerOverflow=off  RndMeth=Floor
  Gain : Gain  Gain=12  OutDataTypeStr=uint16  ParamDataTypeStr=Inherit: Same as input
  Gain1 : Gain  Gain=2  OutDataTypeStr=Inherit: Same as input
  Gain14 : Gain  Gain=8  OutDataTypeStr=Inherit: Same as input
  Gain2 : Gain  Gain=3  OutDataTypeStr=Inherit: Same as input
  Gain3 : Gain  Gain=5  OutDataTypeStr=Inherit: Same as input
  Gain4 : Gain  Gain=6  OutDataTypeStr=Inherit: Same as input
  Gain5 : Gain  Gain=7  OutDataTypeStr=Inherit: Same as input
  Gain6 : Gain  Gain=4  OutDataTypeStr=Inherit: Same as input
  Gain7 : Gain  Gain=9  OutDataTypeStr=Inherit: Same as input
  Gain8 : Gain  Gain=10  OutDataTypeStr=Inherit: Same as input
  Gain9 : Gain  Gain=11  OutDataTypeStr=Inherit: Same as input
  NCO HDL Optimized{1..4,6..13} (12 alike) : dsphdlsigops2/NCO  PhaseIncrementSource=Input port  PhaseIncrement=round(Fo*(2^N)/Fs)  PhaseOffsetSource=Input port  PhaseOffset=0  DitherSource=Property  NumDitherBits=4  SamplesPerFrame=1  LUTCompress=on  ResetAction=off  Waveform=Sine  PhasePort=off  SimulateUsing=Code generation  AccumulatorWL=N  PhaseQuantization=off  NumQuantizerAccumulatorBits=12  OutputDataType=Binary point scaling  OutputWL=14  OutputFL=12
  Subsystem : Subsystem
  Terminator{,1..11} (12 alike) : Terminator
  Vector Concatenate : Concatenate  NumInputs=12
  NCO_Vector_DAC0 : Outport  VectorParamsAs1DForOutWhenUnconnected=off
  Valid : Outport  Port=2  VectorParamsAs1DForOutWhenUnconnected=off
  wires:
  Constant3/1 -> NCO HDL Optimized1/2
  Gain2/1 -> NCO HDL Optimized4/2
  Gain1/1 -> NCO HDL Optimized3/2
  Constant/1 -> Valid/1
  NCO HDL Optimized1/1 -> Data Type Conversion/1
  NCO HDL Optimized2/1 -> Data Type Conversion1/1
  NCO HDL Optimized3/1 -> Data Type Conversion2/1
  ScaleCh0/1 -> Subsystem/2(Scale)
  NCO HDL Optimized4/1 -> Data Type Conversion3/1
  NCO HDL Optimized1/2 -> Terminator/1
  NCO HDL Optimized2/2 -> Terminator1/1
  NCO HDL Optimized3/2 -> Terminator2/1
  NCO HDL Optimized4/2 -> Terminator3/1
  Data Type Conversion/1 -> Vector Concatenate/1
  Data Type Conversion1/1 -> Vector Concatenate/2
  Data Type Conversion2/1 -> Vector Concatenate/3
  Data Type Conversion3/1 -> Vector Concatenate/4
  Vector Concatenate/1 -> Subsystem/1(VectorIn)
  Subsystem/1(NCO_Vector_DAC0) -> NCO_Vector_DAC0/1
  Gain7/1 -> NCO HDL Optimized10/2
  NCO HDL Optimized13/1 -> Data Type Conversion8/1
  NCO HDL Optimized7/1 -> Data Type Conversion5/1
  Gain6/1 -> NCO HDL Optimized6/2
  NCO HDL Optimized10/1 -> Data Type Conversion9/1
  NCO HDL Optimized12/2 -> Terminator11/1
  NCO HDL Optimized9/2 -> Terminator7/1
  Constant1/1 -> NCO HDL Optimized2/3, NCO HDL Optimized3/3, NCO HDL Optimized6/3, NCO HDL Optimized7/3, NCO HDL Optimized8/3, NCO HDL Optimized10/3, NCO HDL Optimized12/3, NCO HDL Optimized11/3, NCO HDL Optimized13/3, NCO HDL Optimized9/3, NCO HDL Optimized4/3, NCO HDL Optimized1/3
  Gain8/1 -> NCO HDL Optimized11/2
  NCO HDL Optimized8/2 -> Terminator6/1
  NCO HDL Optimized10/2 -> Terminator9/1
  Gain5/1 -> NCO HDL Optimized9/2
  Gain9/1 -> NCO HDL Optimized12/2
  Gain/1 -> NCO HDL Optimized1/1, NCO HDL Optimized2/1, NCO HDL Optimized6/1, NCO HDL Optimized7/1, NCO HDL Optimized8/1, NCO HDL Optimized9/1, NCO HDL Optimized13/1, NCO HDL Optimized10/1, NCO HDL Optimized12/1, NCO HDL Optimized11/1, NCO HDL Optimized4/1, NCO HDL Optimized3/1
  Gain3/1 -> NCO HDL Optimized7/2
  NCO HDL Optimized6/2 -> Terminator4/1
  NCO HDL Optimized8/1 -> Data Type Conversion6/1
  NCO HDL Optimized7/2 -> Terminator5/1
  NCO HDL Optimized11/2 -> Terminator10/1
  NCO HDL Optimized11/1 -> Data Type Conversion10/1
  NCO HDL Optimized9/1 -> Data Type Conversion7/1
  NCO HDL Optimized13/2 -> Terminator8/1
  NCO HDL Optimized6/1 -> Data Type Conversion4/1
  NCO HDL Optimized12/1 -> Data Type Conversion11/1
  Gain14/1 -> NCO HDL Optimized13/2
  Gain4/1 -> NCO HDL Optimized8/2
  Increment/1 -> Gain2/1, Gain6/1, Gain5/1, Gain7/1, Gain9/1, Gain8/1, Gain14/1, Gain4/1, Gain3/1, Gain1/1, Gain/1, NCO HDL Optimized2/2
  Data Type Conversion11/1 -> Vector Concatenate/12
  Data Type Conversion10/1 -> Vector Concatenate/11
  Data Type Conversion9/1 -> Vector Concatenate/10
  Data Type Conversion8/1 -> Vector Concatenate/9
  Data Type Conversion7/1 -> Vector Concatenate/8
  Data Type Conversion6/1 -> Vector Concatenate/7
  Data Type Conversion5/1 -> Vector Concatenate/6
  Data Type Conversion4/1 -> Vector Concatenate/5

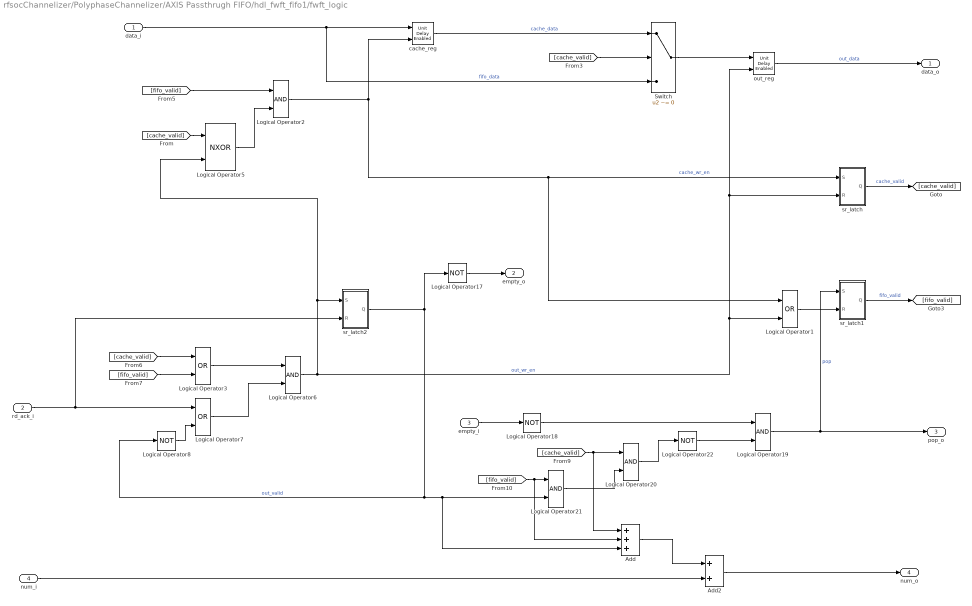
== system rfsocChannelizer/PolyphaseChannelizer/AXIS Passthrugh FIFO/hdl_fwft_fifo1/fwft_logic ==
  data_i : Inport
  rd_ack_i : Inport  Port=2
  empty_i : Inport  Port=3
  num_i : Inport  Port=4
  Add : Sum  Inputs=+++  AccumDataTypeStr=fixdt(0,2,0)
  Add2 : Sum  OutDataTypeStr=fixdt(0,FIFO_CNT_BITS,0)
  Logical Operator1 : Logic  Operator=OR  IconShape=distinctive  AllPortsSameDT=off  OutDataTypeStr=boolean
  Logical Operator{8,17..18,22} (4 alike) : Logic  Operator=NOT  IconShape=distinctive  AllPortsSameDT=off  OutDataTypeStr=boolean
  Logical Operator{2,6,19..21} (5 alike) : Logic  IconShape=distinctive  AllPortsSameDT=off  OutDataTypeStr=boolean
  Logical Operator3 : Logic  Operator=OR  IconShape=distinctive  AllPortsSameDT=off  OutDataTypeStr=boolean
  Logical Operator5 : Logic  Operator=NXOR  IconShape=distinctive  AllPortsSameDT=off  OutDataTypeStr=boolean
  Logical Operator7 : Logic  Operator=OR  IconShape=distinctive  AllPortsSameDT=off  OutDataTypeStr=boolean
  Switch : Switch  Criteria=u2 ~= 0  SaturateOnIntegerOverflow=off  InputSameDT=off
  cache_reg : simulink_need_slupdate/Unit Delay Enabled  vinit=0.0  tsamp=-1
  out_reg : simulink_need_slupdate/Unit Delay Enabled  vinit=0.0  tsamp=-1
  sr_latch : Subsystem
  sr_latch1 : Subsystem
  sr_latch2 : Subsystem
  data_o : Outport  VectorParamsAs1DForOutWhenUnconnected=off
  empty_o : Outport  Port=2  VectorParamsAs1DForOutWhenUnconnected=off
  pop_o : Outport  Port=3  VectorParamsAs1DForOutWhenUnconnected=off
  num_o : Outport  Port=4  VectorParamsAs1DForOutWhenUnconnected=off
  wires:
  empty_i/1 -> Logical Operator18/1
  sr_latch1/1(Q) -> [fifo_valid]  "fifo_valid"
  sr_latch/1(Q) -> [cache_valid]  "cache_valid"
  Switch/1 -> out_reg/1
  data_i/1 -> Switch/3, cache_reg/1  "fifo_data"
  cache_reg/1 -> Switch/1  "cache_data"
  Logical Operator5/1 -> Logical Operator2/2
  Logical Operator6/1 -> Logical Operator5/2, sr_latch2/1(S), out_reg/2, sr_latch/2(R), Logical Operator1/2  "out_wr_en"
  [cache_valid] -> Logical Operator5/1
  [cache_valid] -> Switch/2
  Logical Operator2/1 -> cache_reg/2, Logical Operator1/1, sr_latch/1(S)  "cache_wr_en"
  [fifo_valid] -> Logical Operator2/1
  [cache_valid] -> Logical Operator3/1
  [fifo_valid] -> Logical Operator3/2
  Logical Operator3/1 -> Logical Operator6/1
  Logical Operator7/1 -> Logical Operator6/2
  rd_ack_i/1 -> sr_latch2/2(R), Logical Operator7/1
  sr_latch2/1(Q) -> Logical Operator8/1, Add/3, Logical Operator21/2, Logical Operator17/1  "out_valid"
  Logical Operator8/1 -> Logical Operator7/2
  Logical Operator17/1 -> empty_o/1
  Logical Operator18/1 -> Logical Operator19/1
  Logical Operator21/1 -> Logical Operator20/2
  Logical Operator22/1 -> Logical Operator19/2
  Logical Operator20/1 -> Logical Operator22/1
  Logical Operator19/1 -> pop_o/1, sr_latch1/1(S)  "pop"
  [cache_valid] -> Add/1, Logical Operator20/1
  [fifo_valid] -> Add/2, Logical Operator21/1
  Logical Operator1/1 -> sr_latch1/2(R)
  out_reg/1 -> data_o/1  "out_data"
  num_i/1 -> Add2/2
  Add/1 -> Add2/1
  Add2/1 -> num_o/1

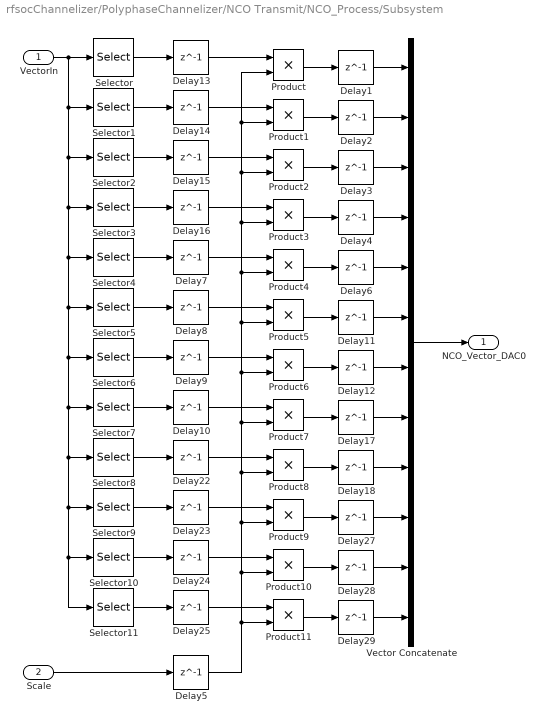
== system rfsocChannelizer/PolyphaseChannelizer/NCO Transmit/NCO_Process/Subsystem ==
  VectorIn : Inport
  Scale : Inport  Port=2
  Delay{1..18,22..25,27..29} (25 alike) : Delay  DelayLength=1
  Product{,1..11} (12 alike) : Product  OutDataTypeStr=Inherit: Same as first input
  Selector : Selector  InputPortWidth=12  IndexOptions=Index vector (dialog)  Indices=1  OutputSizes=1
  Selector1 : Selector  InputPortWidth=12  IndexOptions=Index vector (dialog)  Indices=2  OutputSizes=1
  Selector10 : Selector  InputPortWidth=12  IndexOptions=Index vector (dialog)  Indices=11  OutputSizes=1
  Selector11 : Selector  InputPortWidth=12  IndexOptions=Index vector (dialog)  Indices=12  OutputSizes=1
  Selector2 : Selector  InputPortWidth=12  IndexOptions=Index vector (dialog)  Indices=3  OutputSizes=1
  Selector3 : Selector  InputPortWidth=12  IndexOptions=Index vector (dialog)  Indices=4  OutputSizes=1
  Selector4 : Selector  InputPortWidth=12  IndexOptions=Index vector (dialog)  Indices=5  OutputSizes=1
  Selector5 : Selector  InputPortWidth=12  IndexOptions=Index vector (dialog)  Indices=6  OutputSizes=1
  Selector6 : Selector  InputPortWidth=12  IndexOptions=Index vector (dialog)  Indices=7  OutputSizes=1
  Selector7 : Selector  InputPortWidth=12  IndexOptions=Index vector (dialog)  Indices=8  OutputSizes=1
  Selector8 : Selector  InputPortWidth=12  IndexOptions=Index vector (dialog)  Indices=9  OutputSizes=1
  Selector9 : Selector  InputPortWidth=12  IndexOptions=Index vector (dialog)  Indices=10  OutputSizes=1
  Vector Concatenate : Concatenate  NumInputs=12
  NCO_Vector_DAC0 : Outport  VectorParamsAs1DForOutWhenUnconnected=off
  wires:
  Delay8/1 -> Product5/1
  Delay11/1 -> Vector Concatenate/6
  Delay16/1 -> Product3/1
  Product5/1 -> Delay11/1
  Product10/1 -> Delay28/1
  Delay12/1 -> Vector Concatenate/7
  Delay25/1 -> Product11/1
  Delay4/1 -> Vector Concatenate/4
  Selector6/1 -> Delay9/1
  Delay24/1 -> Product10/1
  Delay7/1 -> Product4/1
  Delay15/1 -> Product2/1
  Selector9/1 -> Delay23/1
  Product3/1 -> Delay4/1
  Delay14/1 -> Product1/1
  Delay3/1 -> Vector Concatenate/3
  Selector10/1 -> Delay24/1
  Product1/1 -> Delay2/1
  Delay13/1 -> Product/1
  Delay18/1 -> Vector Concatenate/9
  Delay10/1 -> Product7/1
  Delay23/1 -> Product9/1
  Selector8/1 -> Delay22/1
  Selector1/1 -> Delay14/1
  Delay9/1 -> Product6/1
  Selector2/1 -> Delay15/1
  Product7/1 -> Delay17/1
  Delay22/1 -> Product8/1
  Delay28/1 -> Vector Concatenate/11
  Delay29/1 -> Vector Concatenate/12
  Product11/1 -> Delay29/1
  Product6/1 -> Delay12/1
  Scale/1 -> Delay5/1
  Delay6/1 -> Vector Concatenate/5
  Selector/1 -> Delay13/1
  Delay2/1 -> Vector Concatenate/2
  Selector4/1 -> Delay7/1
  Product2/1 -> Delay3/1
  Selector5/1 -> Delay8/1
  Product8/1 -> Delay18/1
  Product9/1 -> Delay27/1
  Selector7/1 -> Delay10/1
  Delay27/1 -> Vector Concatenate/10
  Delay5/1 -> Product11/2, Product10/2, Product5/2, Product/2, Product1/2, Product2/2, Product3/2, Product4/2, Product6/2, Product7/2, Product8/2, Product9/2
  Product/1 -> Delay1/1
  Selector3/1 -> Delay16/1
  VectorIn/1 -> Selector8/1, Selector11/1, Selector10/1, Selector9/1, Selector7/1, Selector6/1, Selector5/1, Selector4/1, Selector3/1, Selector2/1, Selector1/1, Selector/1
  Selector11/1 -> Delay25/1
  Product4/1 -> Delay6/1
  Vector Concatenate/1 -> NCO_Vector_DAC0/1
  Delay1/1 -> Vector Concatenate/1
  Delay17/1 -> Vector Concatenate/8

== system rfsocChannelizer/PolyphaseChannelizer/AXIS Passthrugh FIFO/hdl_fwft_fifo1/fwft_logic/sr_latch ==
  S : Inport
  R : Inport  Port=2
  Logical Operator1 : Logic  IconShape=distinctive  AllPortsSameDT=off  OutDataTypeStr=boolean
  Logical Operator2 : Logic  Operator=NOT  IconShape=distinctive  AllPortsSameDT=off  OutDataTypeStr=boolean
  Logical Operator9 : Logic  Operator=OR  IconShape=distinctive  AllPortsSameDT=off  OutDataTypeStr=boolean
  Unit Delay1 : UnitDelay  SampleTime=-1  HasFrameUpgradeWarning=on
  Q : Outport  VectorParamsAs1DForOutWhenUnconnected=off
  wires:
  S/1 -> Logical Operator9/1
  R/1 -> Logical Operator2/1
  Logical Operator2/1 -> Logical Operator1/1
  Unit Delay1/1 -> Logical Operator1/2, Q/1
  Logical Operator9/1 -> Unit Delay1/1
  Logical Operator1/1 -> Logical Operator9/2

== system rfsocChannelizer/PolyphaseChannelizer/AXIS Passthrugh FIFO/hdl_fwft_fifo1/fwft_logic/sr_latch1 ==
  S : Inport
  R : Inport  Port=2
  Logical Operator1 : Logic  IconShape=distinctive  AllPortsSameDT=off  OutDataTypeStr=boolean
  Logical Operator2 : Logic  Operator=NOT  IconShape=distinctive  AllPortsSameDT=off  OutDataTypeStr=boolean
  Logical Operator9 : Logic  Operator=OR  IconShape=distinctive  AllPortsSameDT=off  OutDataTypeStr=boolean
  Unit Delay1 : UnitDelay  SampleTime=-1  HasFrameUpgradeWarning=on
  Q : Outport  VectorParamsAs1DForOutWhenUnconnected=off
  wires:
  Logical Operator1/1 -> Logical Operator9/2
  Logical Operator9/1 -> Unit Delay1/1
  Unit Delay1/1 -> Q/1, Logical Operator1/2
  Logical Operator2/1 -> Logical Operator1/1
  R/1 -> Logical Operator2/1
  S/1 -> Logical Operator9/1

== system rfsocChannelizer/PolyphaseChannelizer/AXIS Passthrugh FIFO/hdl_fwft_fifo1/fwft_logic/sr_latch2 ==
  S : Inport
  R : Inport  Port=2
  Logical Operator1 : Logic  IconShape=distinctive  AllPortsSameDT=off  OutDataTypeStr=boolean
  Logical Operator2 : Logic  Operator=NOT  IconShape=distinctive  AllPortsSameDT=off  OutDataTypeStr=boolean
  Logical Operator9 : Logic  Operator=OR  IconShape=distinctive  AllPortsSameDT=off  OutDataTypeStr=boolean
  Unit Delay1 : UnitDelay  SampleTime=-1  HasFrameUpgradeWarning=on
  Q : Outport  VectorParamsAs1DForOutWhenUnconnected=off
  wires:
  S/1 -> Logical Operator9/1
  R/1 -> Logical Operator2/1
  Logical Operator2/1 -> Logical Operator1/1
  Unit Delay1/1 -> Logical Operator1/2, Q/1
  Logical Operator9/1 -> Unit Delay1/1
  Logical Operator1/1 -> Logical Operator9/2

== matlab function rfsocChannelizer/PolyphaseChannelizer/Channelizer Receive Processing /MATLAB Function ==
  data: trigger input; sof_i input; valid_i input; FFTSize input; ready input; valid_o output; tlast_o output
function [valid_o,tlast_o] = FFT_Capture(trigger,sof_i,valid_i,FFTSize,ready)
persistent state counter

WAIT_ON_TRIGGER = uint8(0);
WAIT_ON_SOF = uint8(1);
WRITE_FRAME = uint8(2);
valid_o = false;
tlast_o = false;

if isempty(state)
    state = WAIT_ON_TRIGGER;
    counter = uint32(0);
end

switch(state)
    case(WAIT_ON_TRIGGER)
        counter(:) = 0;
        if trigger && ready && ~sof_i            
            state(:) = WAIT_ON_SOF;
        elseif trigger && ready && sof_i  
            % jump immediatley to WRITE_FRAME            
            counter(:) = counter(:) + 1;
            valid_o = true;
            state(:) = WRITE_FRAME;        
        end        
    case(WAIT_ON_SOF)
        if sof_i && valid_i             
            state(:) = WRITE_FRAME;
            counter(:) = counter(:) + 1;
            valid_o = true;
        end
    case(WRITE_FRAME)
        if valid_i
            if counter < FFTSize-1
                counter(:) = counter(:) + 1;
                valid_o = true;
            elseif counter == FFTSize - 1
                counter(:) = counter(:) + 1;
                tlast_o = true;
                valid_o = true;
            else
                counter(:) = 0;
                state(:) = WAIT_ON_TRIGGER;
            end
        end
        
end

== matlab function rfsocChannelizer/DMA_Representation ==
  data: newFrameTrigger output; u input; Frame output; valid input; tlast input
function [newFrameTrigger,Frame] = fcn(u,valid,tlast)

persistent StoreArray idx
frameSize = 512;
if isempty(StoreArray)
    StoreArray = cast(zeros(frameSize,1),'like',u);
    idx = uint32(1);
end


if valid && idx <= frameSize
    StoreArray(idx)   = u;
%     StoreArray(idx+1) = u(2);
%     StoreArray(idx+2) = u(3);
%     StoreArray(idx+3) = u(4);
    idx = idx + 1;
end

if tlast %equivilant to TLAST
    if idx ~= (frameSize + 1)
        disp(strcat('TLAST finished early: ', num2str(frameSize)));
    end    
    idx(:) = 1;    
    newFrameTrigger = true;
    
    Frame = StoreArray;
    
else
    newFrameTrigger = false;
    Frame = StoreArray;
end
